simulink model "nonLinearSingleTrack_SchrammHiller"  (R2018b)
settings: Solver=VariableStepAuto  StartTime=0.0  StopTime=10.0  RelTol=1e-3
settings Model: Creator=utente  LastModifiedBy=utente

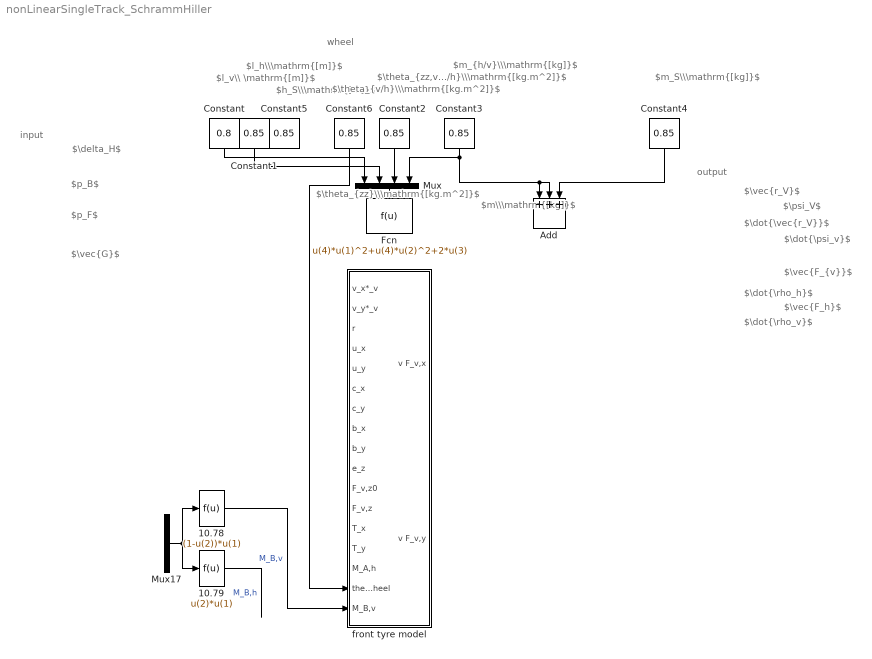
== system nonLinearSingleTrack_SchrammHiller ==
  note: wheel
  note: $l_v\\ \mathrm{[m]}$
  note: output
  note: $\vec{F_h}$
  note: $\vec{F_{v}}$
  note: $\dot{\rho_h}$
  note: $\dot{\rho_v}$
  note: $\dot{\psi_v}$
  note: $\psi_V$
  note: $\dot{\vec{r_V}}$
  note: $\vec{r_V}$
  note: input
  note: $\vec{G}$
  note: $p_B$
  note: $p_F$
  note: $\delta_H$
  note: $l_h\\\mathrm{[m]}$
  note: $\theta_{zz,v/h}\\\mathrm{[kg.m^2]}$
  note: $m_{h/v}\\\mathrm{[kg]}$
  note: $m_S\\\mathrm{[kg]}$
  note: $m\\\mathrm{[kg]}$
  note: $h_S\\\mathrm{[m]}$
  note: $\theta_{zz}\\\mathrm{[kg.m^2]}$
  note: $\theta_{v/h}\\\mathrm{[kg.m^2]}$
  10.78 : Fcn  Expr=(1-u(2))*u(1)
  10.79 : Fcn  Expr=u(2)*u(1)
  Add : Sum  Inputs=+++
  Constant : Constant  Value=0.8
  Constant{1..6} (6 alike) : Constant  Value=0.85
  Fcn : Fcn  Expr=u(4)*u(1)^2+u(4)*u(2)^2+2*u(3)
  Mux : Mux
  Mux17 : Mux  Inputs=2
  front tyre model : Subsystem
  wires:
  Constant3/1 -> Mux/4, Add/2, Add/1
  Constant4/1 -> Add/3
  Mux/1 -> Fcn/1
  Constant2/1 -> Mux/3
  Constant/1 -> Mux/1
  Constant1/1 -> Mux/2
  ? -> Mux17/1  "M_B"
  ? -> Mux17/2  "xi_b"
  10.78/1 -> front tyre model/17(M_B,v)  "M_B,v"
  Mux17/1 -> 10.79/1, 10.78/1
  10.79/1 -> ?  "M_B,h"
  Constant6/1 -> front tyre model/16(theta_wheel)

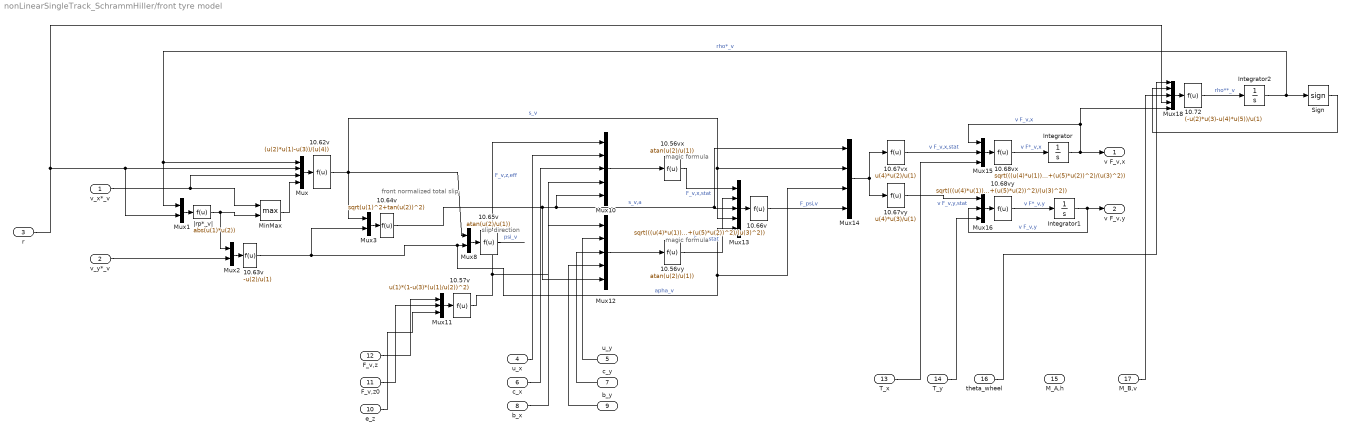
== system nonLinearSingleTrack_SchrammHiller/front tyre model ==
  note: slip direction
  note: front normalized
      | total slip
  note: magic formula
  note: magic formula
  v_x*_v : Inport
  v_y*_v : Inport  Port=2
  r : Inport  Port=3
  u_x : Inport  Port=4
  u_y : Inport  Port=5
  c_x : Inport  Port=6
  c_y : Inport  Port=7
  b_x : Inport  Port=8
  b_y : Inport  Port=9
  e_z : Inport  Port=10
  F_v,z0 : Inport  Port=11
  F_v,z : Inport  Port=12
  T_x : Inport  Port=13
  T_y : Inport  Port=14
  M_A,h : Inport  Port=15
  theta_wheel : Inport  Port=16
  M_B,v : Inport  Port=17
  10.56vx : Fcn  Expr=atan(u(2)/u(1))
  10.56vy : Fcn  Expr=atan(u(2)/u(1))
  10.57v : Fcn  Expr=u(1)*(1-u(3)*(u(1)/u(2))^2)
  10.62v : Fcn  Expr=(u(2)*u(1)-u(3))/(u(4))
  10.63v : Fcn  Expr=-u(2)/u(1)
  10.64v : Fcn  Expr=sqrt(u(1)^2+tan(u(2))^2)
  10.65v : Fcn  Expr=atan(u(2)/u(1))
  10.66v : Fcn  Expr=sqrt(((u(4)*u(1))^2+(u(5)*u(2))^2)/(u(3)^2))
  10.67vx : Fcn  Expr=u(4)*u(2)/u(1)
  10.67vy : Fcn  Expr=u(4)*u(3)/u(1)
  10.68vx : Fcn  Expr=sqrt(((u(4)*u(1))^2+(u(5)*u(2))^2)/(u(3)^2))
  10.68vy : Fcn  Expr=sqrt(((u(4)*u(1))^2+(u(5)*u(2))^2)/(u(3)^2))
  10.72 : Fcn  Expr=(-u(2)*u(3)-u(4)*u(5))/u(1)
  Integrator : Integrator
  Integrator1 : Integrator
  Integrator2 : Integrator
  MinMax : MinMax  Function=max  Inputs=2
  Mux : Mux
  Mux{1..3,8} (4 alike) : Mux  Inputs=2
  Mux{10,12..13,18} (4 alike) : Mux  Inputs=5
  Mux11 : Mux  Inputs=3
  Mux14 : Mux
  Mux15 : Mux  Inputs=3
  Mux16 : Mux  Inputs=3
  Sign : Signum
  "|rp*_v| " : Fcn  Expr=abs(u(1)*u(2))
  v F_v,x : Outport
  v F_v,y : Outport  Port=2
  wires:
  Mux/1 -> 10.62v/1
  v_x*_v/1 -> MinMax/1, Mux/3
  Mux1/1 -> "|rp*_v| "/1
  "|rp*_v| "/1 -> Mux2/1, MinMax/2
  MinMax/1 -> Mux/4
  Mux2/1 -> 10.63v/1
  v_y*_v/1 -> Mux2/2
  Mux3/1 -> 10.64v/1
  10.64v/1 -> Mux12/5, Mux10/5, Mux14/1, Mux13/3  "s_v,a"
  r/1 -> Mux1/2, Mux/2, Mux18/4
  10.65v/1 -> ?  "psi_v"
  Mux8/1 -> 10.65v/1
  10.63v/1 -> Mux14/3, Mux13/5, Mux8/2, Mux3/2  "apha_v"
  Mux10/1 -> 10.56vx/1
  10.56vx/1 -> Mux13/1  "F_v,x,stat"
  u_x/1 -> Mux10/2
  c_x/1 -> Mux10/3
  b_x/1 -> Mux10/4
  F_v,z/1 -> Mux11/1
  F_v,z0/1 -> Mux11/2
  e_z/1 -> Mux11/3
  Mux11/1 -> 10.57v/1
  10.57v/1 -> Mux12/1, Mux10/1  "F_v,z,eff"
  10.56vy/1 -> Mux13/2  "F_v,y,stat"
  Mux12/1 -> 10.56vy/1
  u_y/1 -> Mux12/2
  c_y/1 -> Mux12/3
  b_y/1 -> Mux12/4
  10.62v/1 -> Mux3/1, Mux14/2, Mux13/4, Mux8/1  "s_v"
  Mux13/1 -> 10.66v/1
  10.66v/1 -> Mux14/4  "F_psi,v"
  Mux14/1 -> 10.67vx/1, 10.67vy/1
  10.67vx/1 -> Mux15/2  "v F_v,x,stat"
  10.67vy/1 -> Mux16/1  "v F_v,y,stat"
  Integrator/1 -> v F_v,x/1, Mux18/5, Mux15/1  "v F_v,x"
  Mux15/1 -> 10.68vx/1
  Mux16/1 -> 10.68vy/1
  10.68vx/1 -> Integrator/1  "v F*_v,x"
  10.68vy/1 -> Integrator1/1  "v F*_v,y"
  Integrator1/1 -> v F_v,y/1, Mux16/2  "v F_v,y"
  T_x/1 -> Mux15/3
  T_y/1 -> Mux16/3
  Integrator2/1 -> Mux1/1, Mux/1, Sign/1  "rho*_v"
  Mux18/1 -> 10.72/1
  10.72/1 -> Integrator2/1  "rho**_v"
  theta_wheel/1 -> Mux18/1
  Sign/1 -> Mux18/2
  M_B,v/1 -> Mux18/3
